simulink model "pendModelSimulink"  (R2023b)
settings: Solver=VariableStepAuto  StartTime=0.0  StopTime=20  RelTol=1e-3
values from neighbouring files (symbols this model uses):
  A = [0      1              0           0 ... (first row only)    [pendModel_SS.m]    (also in settlingTimeAnalysis.m)
  B = [     0 ... (first row only)    [pendModel_SS.m]    (also in settlingTimeAnalysis.m)
  C = [1 0 0 0 ... (first row only)    [pendModel_SS.m]    (also in settlingTimeAnalysis.m)
  K_lqr = lqr(A,B,Q,R)    [pendModel_SS.m]    (also in settlingTimeAnalysis.m)
  x0 = [0; -5*pi/180; 0; 0]    [pendModel_SS.m]    (also in settlingTimeAnalysis.m)
settings Model: Creator=mattp  LastModifiedBy=mattp

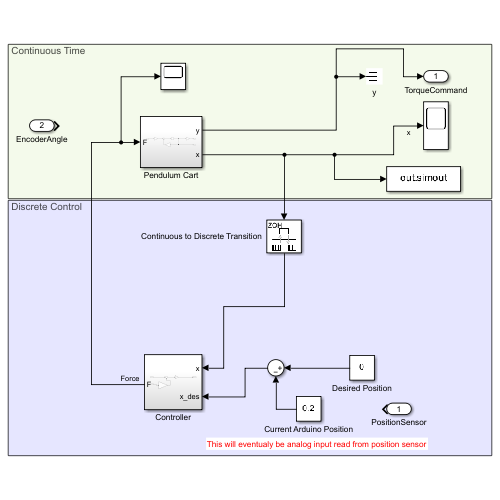
[thumbnail: Simulink's stored preview of the top-level diagram]
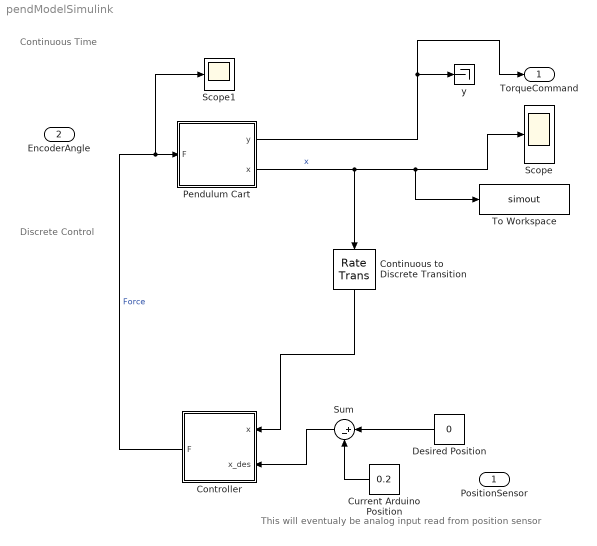
== system pendModelSimulink ==
  note: This will eventualy be analog input read from position sensor
  note: Continuous Time
  note: Discrete Control
  PositionSensor : Inport
  EncoderAngle : Inport  Port=2
  Continuous to Discrete Transition : RateTransition  OutPortSampleTime=.05
  Controller : Subsystem
  Current Arduino Position : Constant  Value=0.2
  Desired Position : Constant  Value=0
  Pendulum Cart : Subsystem
  Scope : Scope
  Scope1 : Scope
  Sum : Sum  Inputs=|+-
  To Workspace : ToWorkspace  VariableName=simout  SaveFormat=Timeseries  SampleTime=-1
  y : Terminator
  TorqueCommand : Outport
  wires:
  Pendulum Cart/1(y) -> TorqueCommand/1, y/1
  Pendulum Cart/2(x) -> Scope/1, To Workspace/1, Continuous to Discrete Transition/1  "x"
  Desired Position/1 -> Sum/1
  Current Arduino Position/1 -> Sum/2
  Controller/1(F) -> Scope1/1, Pendulum Cart/1(F)  "Force"
  Sum/1 -> Controller/2(x_des)
  Continuous to Discrete Transition/1 -> Controller/1(x)

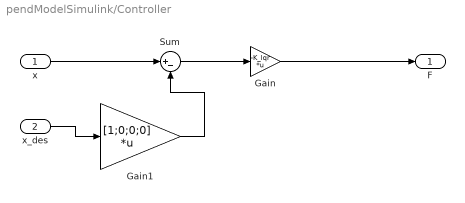
== system pendModelSimulink/Controller ==
  x : Inport
  x_des : Inport  Port=2
  Gain : Gain  Gain=-K_lqr  Multiplication=Matrix(K*u)
  Gain1 : Gain  Gain=[1;0;0;0]  Multiplication=Matrix(K*u)
  Sum : Sum  Inputs=|+-
  F : Outport
  wires:
  x/1 -> Sum/1
  Gain/1 -> F/1
  x_des/1 -> Gain1/1
  Gain1/1 -> Sum/2
  Sum/1 -> Gain/1

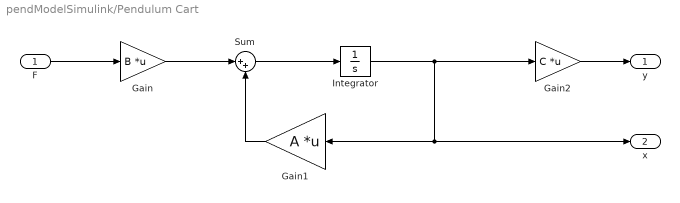
== system pendModelSimulink/Pendulum Cart ==
  F : Inport
  Gain : Gain  Gain=B  Multiplication=Matrix(K*u)
  Gain1 : Gain  Gain=A  Multiplication=Matrix(K*u) (u vector)
  Gain2 : Gain  Gain=C  Multiplication=Matrix(K*u)
  Integrator : Integrator  InitialCondition=x0
  Sum : Sum  Inputs=|++
  y : Outport
  x : Outport  Port=2
  wires:
  Integrator/1 -> x/1, Gain1/1, Gain2/1
  F/1 -> Gain/1
  Gain1/1 -> Sum/2
  Sum/1 -> Integrator/1
  Gain2/1 -> y/1
  Gain/1 -> Sum/1
